simulink model "resistenciaBacteriasSal1_entrada"  (R2018a)
settings: Solver=VariableStepAuto  StartTime=0.0  StopTime=800  MaxStep=0.05  RelTol=1e-3
values from neighbouring files (symbols this model uses):
  ro = 0.0683    [LaplaceAzeta.m]    (also in discretizacion.m = 0.0683238685925)
  so = 0.3356    [LaplaceAzeta.m]    (also in discretizacion.m = 0.335599308431)
settings Model: Creator=posoriol1  LastModifiedBy=posoriol1
settings CodeAppCC: StateflowObjectComments=on

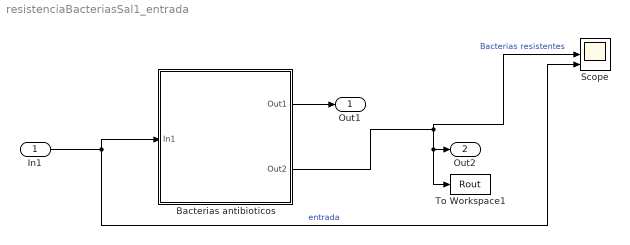
== system resistenciaBacteriasSal1_entrada ==
  In1 : Inport
  Bacterias antibioticos : Subsystem  mask{par=[0.4,0.1,0.3960,4^(-3),0.2,0.09,0.0083], x0=[so,ro]}
      mask prompts: par "[bs br alphas q ms mr mc]"; x0 "Cond iniciales (s0,r0)"
      mask init:
      | bs=par(1);br=par(2);alphas=par(3);q=par(4);ms=par(5);mr=par(6);mc=par(7);
      mask Display: image(imread('bacteria.jpeg'))
  Scope : Scope  NumInputPorts=3
  To Workspace1 : ToWorkspace  VariableName=Rout  SampleTime=-1
  Out1 : Outport
  Out2 : Outport  Port=2
  wires:
  In1/1 -> Bacterias antibioticos/1(In1), Scope/3  "entrada"
  Bacterias antibioticos/2(Out2) -> Scope/2, Out2/1, To Workspace1/1  "Bacterias resistentes"
  Bacterias antibioticos/1(Out1) -> Out1/1

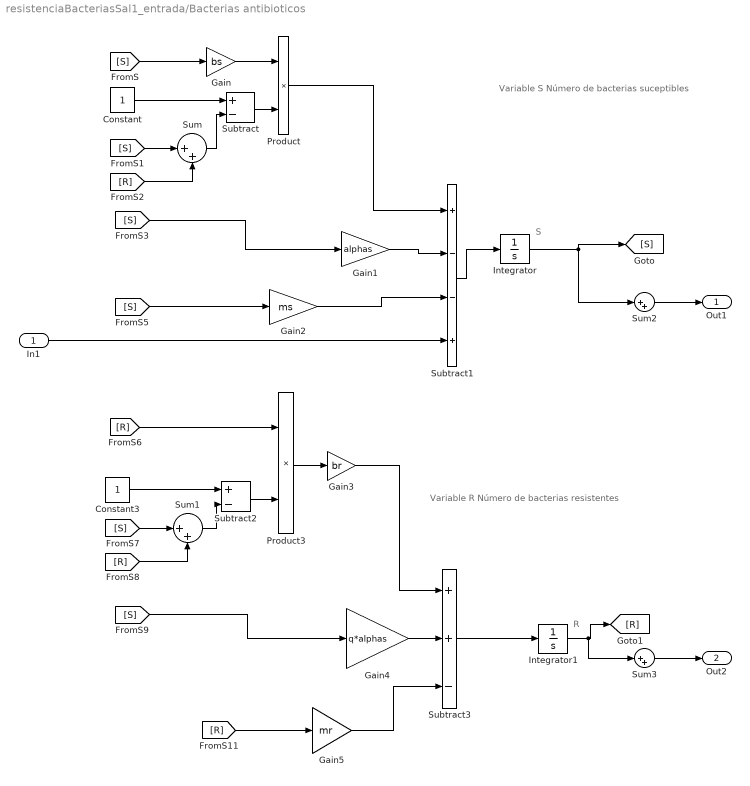
== system resistenciaBacteriasSal1_entrada/Bacterias antibioticos ==
  note: R
  note: S
  note: Variable S
      | Número de bacterias suceptibles
  note: Variable R
      | Número de bacterias resistentes
  In1 : Inport
  Constant : Constant
  Constant3 : Constant
  Gain : Gain  Gain=bs
  Gain1 : Gain  Gain=alphas
  Gain2 : Gain  Gain=ms
  Gain3 : Gain  Gain=br
  Gain4 : Gain  Gain=q*alphas
  Gain5 : Gain  Gain=mr
  Integrator : Integrator  InitialCondition=x0(1)
  Integrator1 : Integrator  InitialCondition=x0(2)
  Product : Product
  Product3 : Product
  Subtract : Sum  Inputs=+-
  Subtract1 : Sum  Inputs=+--+
  Subtract2 : Sum  Inputs=+-
  Subtract3 : Sum  Inputs=++-
  Sum{,1..3} (4 alike) : Sum  Inputs=|++
  Out1 : Outport
  Out2 : Outport  Port=2
  wires:
  [S] -> Sum/1
  [R] -> Sum/2
  Constant/1 -> Subtract/1
  [S] -> Sum1/1
  Sum1/1 -> Subtract2/2
  Subtract1/1 -> Integrator/1
  Integrator/1 -> [S], Sum2/1
  [R] -> Sum1/2
  Constant3/1 -> Subtract2/1
  Product3/1 -> Gain3/1
  Product/1 -> Subtract1/1
  Integrator1/1 -> Sum3/1, [R]
  Subtract3/1 -> Integrator1/1
  Sum/1 -> Subtract/2
  [S] -> Gain/1
  Gain/1 -> Product/1
  Subtract/1 -> Product/2
  [S] -> Gain1/1
  Gain1/1 -> Subtract1/2
  [S] -> Gain2/1
  Gain2/1 -> Subtract1/3
  Gain3/1 -> Subtract3/1
  [R] -> Product3/1
  Subtract2/1 -> Product3/2
  Gain4/1 -> Subtract3/2
  [S] -> Gain4/1
  Gain5/1 -> Subtract3/3
  [R] -> Gain5/1
  In1/1 -> Subtract1/4
  Sum3/1 -> Out2/1
  Sum2/1 -> Out1/1
